simulink model "Aufgabe2_1"  (Simulink 9.1)
settings: Solver=VariableStepAuto  StartTime=0.0  StopTime=10.0  RelTol=1e-3
InitFcn:
  | run('Auf2_1_Initialisierung.m') % Initialisierung
values from neighbouring files (symbols this model uses):
  b1 = 2.39e6    (= 2390000)    [Auf2_1_Initialisierung.m]
  coe = 36.5e6    (= 36500000)    [Auf2_1_Initialisierung.m]
  cp = 75e6    (= 75000000)    [Auf2_1_Initialisierung.m]
  mg = mp + mk    (= 268.7)    [Auf2_1_Initialisierung.m]
settings Model: Creator=kleist  LastModifiedBy=kleist
settings DataIOCC: SaveFormat=Dataset
settings OptimizationCC: LifeSpan=auto
settings DebuggingCC: UnderspecifiedInitializationDetection=Simplified  MergeDetectMultiDrivingBlocksExec=error  SFUnexpectedBacktrackingDiag=error  SFNoUnconditionalDefaultTransitionDiag=error  SFExecutionAtInitializationDiag=warning
settings HardwareCC: ProdBitPerPointer=64  ProdBitPerSizeT=64  ProdBitPerPtrDiffT=64  ProdLargestAtomicFloat=Float  ProdIntDivRoundTo=Zero  ProdEndianess=LittleEndian  ProdWordSize=64  ProdHWDeviceType=Intel->x86-64 (Windows64)
settings ModelReferenceCC: PropagateSignalLabelsOutOfModel=on
settings CodeAppCC: StateflowObjectComments=off
settings GRTTargetCC: TargetLangStandard=C99 (ISO)  CombineOutputUpdateFcns=on  GRTInterface=off
settings ConfigComp: CovMetricSettings=dwe  CovHtmlReporting=off  CovSaveCumulativeToWorkspaceVar=off  CovSaveSingleToWorkspaceVar=off  CovExternalEMLEnable=on

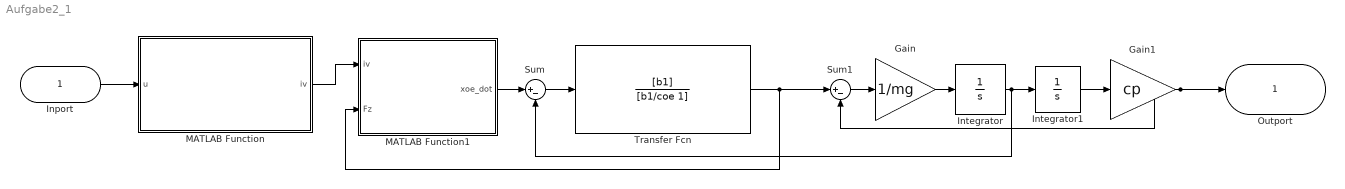
== system Aufgabe2_1 ==
  Inport : Inport
  Gain : Gain  Gain=1/mg
  Gain1 : Gain  Gain=cp
  Integrator : Integrator
  Integrator1 : Integrator
  MATLAB Function : MATLAB Function  TreatAsAtomicUnit=on
  MATLAB Function1 : MATLAB Function  TreatAsAtomicUnit=on
  Sum : Sum  Inputs=|+-
  Sum1 : Sum  Inputs=|+-
  Transfer Fcn : TransferFcn  Numerator=[b1]  Denominator=[b1/coe 1]
  Outport : Outport
  wires:
  Inport/1 -> MATLAB Function/1(u)
  MATLAB Function/1(iv) -> MATLAB Function1/1(iv)
  MATLAB Function1/1(xoe_dot) -> Sum/1
  Sum/1 -> Transfer Fcn/1
  Transfer Fcn/1 -> Sum1/1, MATLAB Function1/2(Fz)
  Sum1/1 -> Gain/1
  Gain/1 -> Integrator/1
  Integrator/1 -> Sum/2, Integrator1/1
  Integrator1/1 -> Gain1/1
  Gain1/1 -> Sum1/2, Outport/1

== matlab function MATLAB Function1 ==
  data: iv input double; xoe_dot output double; Fz input double
function xoe_dot = fcn(iv,Fz)
Ksv = 0.796;%[m/As]
FN = 63000;%[N]
A = 1-Fz/FN*sign(iv);
if A > 0
    xoe_dot = iv*Ksv*sqrt(A);
else
    xoe_dot = 0;
end

== matlab function MATLAB Function ==
  settings: updateMethod=DISCRETE
  data: u input double; iv output double; ivmax data_store_memory double; Kl data_store_memory double
function iv = fcn(u)
Kl = 1; %[A/V]
ivmax = 1;%[A]
if u>1
    iv = ivmax;
elseif u>=-1 &&u<=1
    iv = Kl*u;
else
    iv = -ivmax;
end
